simulink model "Quadcopter_dynamics_simulation"  (R2020a)
settings: Solver=VariableStepAuto  StartTime=0.0  StopTime=inf  RelTol=1e-3
libraries: vrlib x1, sharedtransform x1, robotuavlib x1
settings Model: Creator=rupam  LastModifiedBy=rupam

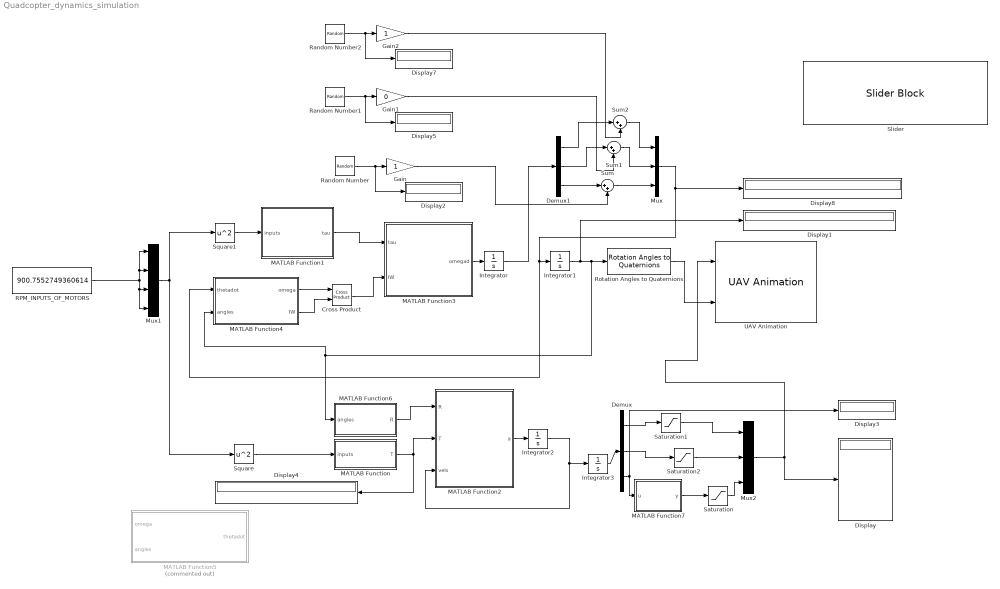
== system Quadcopter_dynamics_simulation ==
  Cross Product : vrlib/Utilities/Cross Product
  Demux : Demux  Outputs=3
  Demux1 : Demux  Outputs=3
  Display{,1..5,7..8} (8 alike) : Display
  Gain : Gain
  Gain1 : Gain  Gain=0
  Gain2 : Gain
  Integrator{,1..3} (4 alike) : Integrator
  MATLAB Function : MATLAB Function  TreatAsAtomicUnit=on
  MATLAB Function1 : MATLAB Function  TreatAsAtomicUnit=on
  MATLAB Function2 : MATLAB Function  TreatAsAtomicUnit=on
  MATLAB Function3 : MATLAB Function  TreatAsAtomicUnit=on
  MATLAB Function4 : MATLAB Function  TreatAsAtomicUnit=on
  MATLAB Function5 : MATLAB Function  Commented=on  TreatAsAtomicUnit=on
  MATLAB Function6 : MATLAB Function  TreatAsAtomicUnit=on
  MATLAB Function7 : MATLAB Function  TreatAsAtomicUnit=on
  Mux : Mux  Inputs=3
  Mux1 : Mux
  Mux2 : Mux  Inputs=3
  RPM_INPUTS_OF_MOTORS : Constant  Value=900.7552749360614
  Random Number : RandomNumber
  Random Number1 : RandomNumber
  Random Number2 : RandomNumber
  Rotation Angles to Quaternions : sharedtransform/Rotation Angles to Quaternions  rotationOrder=XYZ  aMode=aMode
      settings: SourceProductBaseCode=AE,PW,MT,VE,VP
  Saturation : Saturate  UpperLimit=5
  Saturation1 : Saturate  UpperLimit=100  LowerLimit=-100
  Saturation2 : Saturate  UpperLimit=100  LowerLimit=100
  Slider : SliderBlock  ScaleMax=1500
  Square : Math  Operator=square  SaturateOnIntegerOverflow=on
  Square1 : Math  Operator=square  SaturateOnIntegerOverflow=on
  Sum : Sum  Inputs=|++
  Sum1 : Sum  Inputs=|++
  Sum2 : Sum  Inputs=|++
  UAV Animation : robotuavlib/UAV Animation  UAVType=Multirotor  UAVSize=1  InertialZDirection=Up  SampleTime=-1
      settings: SourceProductBaseCode=ROBOTICS_UAV_LIB
  wires:
  MATLAB Function1/1(tau) -> MATLAB Function3/1(tau)
  MATLAB Function/1(T) -> Display4/1, MATLAB Function2/2(T)
  MATLAB Function6/1(R) -> MATLAB Function2/1(R)
  MATLAB Function2/1(a) -> Integrator2/1
  Integrator2/1 -> MATLAB Function2/3(vels), Integrator3/1
  MATLAB Function3/1(omegad) -> Integrator/1
  MATLAB Function4/1(omega) -> Cross Product/1
  Cross Product/1 -> MATLAB Function3/2(IW)
  MATLAB Function4/2(IW) -> Cross Product/2
  Integrator1/1 -> Display1/1, Rotation Angles to Quaternions/1, MATLAB Function6/1(angles), MATLAB Function4/2(angles)
  Integrator3/1 -> Demux/1
  RPM_INPUTS_OF_MOTORS/1 -> Mux1/1, Mux1/2, Mux1/4, Mux1/3
  Mux1/1 -> Square/1, Square1/1
  Square/1 -> MATLAB Function/1(inputs)
  Square1/1 -> MATLAB Function1/1(inputs)
  Demux/3 -> MATLAB Function7/1(u), Display3/1
  Demux/1 -> Saturation1/1
  Demux/2 -> Saturation2/1
  MATLAB Function7/1(y) -> Saturation/1
  Mux2/1 -> UAV Animation/1, Display/1
  Rotation Angles to Quaternions/1 -> UAV Animation/2
  Saturation/1 -> Mux2/3
  Integrator/1 -> Demux1/1
  Gain/1 -> Sum/2
  Random Number/1 -> Display2/1, Gain/1
  Mux/1 -> MATLAB Function4/1(thetadot), Integrator1/1, Display8/1
  Sum1/1 -> Mux/2
  Random Number1/1 -> Display5/1, Gain1/1
  Gain1/1 -> Sum1/2
  Sum2/1 -> Mux/1
  Random Number2/1 -> Display7/1, Gain2/1
  Gain2/1 -> Sum2/2
  Sum/1 -> Mux/3
  Demux1/1 -> Sum2/1
  Demux1/2 -> Sum1/1
  Demux1/3 -> Sum/1
  Saturation1/1 -> Mux2/1
  Saturation2/1 -> Mux2/2

== matlab function Quadcopter_dynamics_simulation/MATLAB Function1 ==
  data: inputs input; tau output
% Compute torques, given current inputs, length, drag coefficient, and thrust coefficient.
function tau = torques(inputs)
    g = 9.81;
    m = 0.5;
    L = 0.25;
    k = 3e-6;
    b = 1e-7;
    I = diag([5e-3, 5e-3, 10e-3]);
    kd = 0.25;
    
tau = [
        L * k * (inputs(1) - inputs(3))
        L * k * (inputs(2) - inputs(4))
        b * (inputs(1) - inputs(2) + inputs(3) - inputs(4))
    ];
end

== matlab function Quadcopter_dynamics_simulation/MATLAB Function ==
  data: inputs input; T output
function T = thrust(inputs)
       g = 9.81;
    m = 0.5;
    L = 0.25;
    k = 3e-6;
    b = 1e-7;
    I = diag([5e-3, 5e-3, 10e-3]);
    kd = 0.25;
 
    T = [0; 0; k * sum(inputs)];
end

== matlab function Quadcopter_dynamics_simulation/MATLAB Function2 ==
  data: a output; R input; T input; vels input
% Compute acceleration in inertial reference frame
% Parameters:
%   g: gravity acceleration
%   m: mass of quadcopter
%   k: thrust coefficient
%   kd: global drag coefficient
     
function a = acceleration(R,T,vels)
    g = 9.81;
    m = 0.5;
    L = 0.25;
    k = 3e-6;
    b = 1e-7;
    I = diag([5e-3, 5e-3, 10e-3]);
    kd = 0.5;
 
    gravity = [0; 0; -g];
    %R = rotation(angles);
    T1 = (R * T);
    Fd = -kd * vels;
    a = gravity + 1 / m * T1 + Fd;
end

== matlab function Quadcopter_dynamics_simulation/MATLAB Function3 ==
  data: tau input; omegad output; IW input
% Compute angular acceleration in body frame
% Parameters:
%   I: inertia matrix
function omegad = angular_acceleration(tau, IW)
%     g = 9.81;
%     m = 0.5;
%     L = 0.25;
%     k = 3e-6;
%     b = 1e-7;
    I = diag([5e-3 5e-3  10e-3]);
%     kd = 0.25;
    omegad = I\(tau - IW);
end

== matlab function Quadcopter_dynamics_simulation/MATLAB Function4 ==
  data: thetadot input; omega output; angles input; IW output
% Convert derivatives of roll, pitch, yaw to omega.
function [omega,IW]= thetadot2omega(thetadot, angles)
    phi = angles(1);
    theta = angles(2);
    psi = angles(3);
    W = [
        1, 0, -sin(theta);
        0, cos(phi), cos(theta)*sin(phi);
        0, -sin(phi), cos(theta)*cos(phi)];
    omega = W *thetadot;
    I = diag([5e-3 5e-3  10e-3]);
    IW=I*omega;
end

== matlab function Quadcopter_dynamics_simulation/MATLAB Function5 ==
  data: omega input; thetadot output; angles input

% Convert omega to roll, pitch, yaw derivatives
function thetadot = omega2thetadot(omega, angles)
    phi = angles(1);
    theta = angles(2);
    psi = angles(3);
    W = [1, 0, -sin(theta)
         0, cos(phi), cos(theta)*sin(phi)
         0, -sin(phi), cos(theta)*cos(phi)];
    thetadot = W\omega;
end

== matlab function Quadcopter_dynamics_simulation/MATLAB Function6 ==
  data: angles input; R output
function R = rotation(angles)
phi = angles(3);
theta = angles(2);
psi = angles(1);
R = zeros(3);
R(:, 1) = [
cos(phi) * cos(theta)
cos(theta) * sin(phi)
- sin(theta)
];
R(:, 2) = [
cos(phi) * sin(theta) * sin(psi) - cos(psi) * sin(phi)
cos(phi) * cos(psi) + sin(phi) * sin(theta) * sin(psi)
cos(theta) * sin(psi)
];
R(:, 3) = [
sin(phi) * sin(psi) + cos(phi) * cos(psi) * sin(theta)
cos(psi) * sin(phi) * sin(theta) - cos(phi) * sin(psi)
cos(theta) * cos(psi)
];
end

== matlab function Quadcopter_dynamics_simulation/MATLAB Function7 ==
  data: u input; y output
function y = fcn(u)
if(u<0)
    y=0;
else
    y=u';

end
